simulink model "solverex"  (R2022b)
settings: Solver=VariableStepAuto  StartTime=0.0  StopTime=0.9  FixedStep=0.1  MaxStep=0.1  RelTol=1e-3
settings Model: Creator=Brigosha_Guest  LastModifiedBy=Brigosha_Guest
settings DataIOCC: LoadExternalInput=on

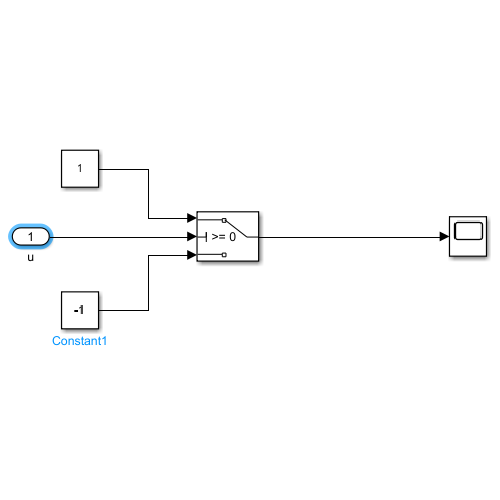
[thumbnail: Simulink's stored preview of the top-level diagram]
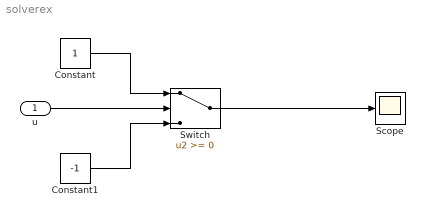
== system solverex ==
  u : Inport
  Constant : Constant
  Constant1 : Constant  Value=-1
  Scope : Scope
  Switch : Switch  SaturateOnIntegerOverflow=off  InputSameDT=off
  wires:
  Constant/1 -> Switch/1
  Constant1/1 -> Switch/3
  u/1 -> Switch/2
  Switch/1 -> Scope/1
